simulink model "test_ic_delta_mapping"  (R2025b)
settings: Solver=FixedStepAuto  StartTime=0.0  StopTime=5  FixedStep=50e-6  RelTol=1e-3
undefined symbols (not defined in the file or in its folder): D_201, delta0_201, M_201, Pe_scale, Pm_201, Pm_step_amp_201, Pm_step_t_201, Vmag_201, VSGScale_201, wn_const
libraries: spsControlledVoltageSourceLib x3, spsSeriesRLCBranchLib x3, spsGroundLib x1, spsThreePhasePISectionLineLib x1, spsThreePhaseVIMeasurementLib x1, spsThreePhaseSourceLib x1, spspowerguiLib x1
settings Model: Creator=27443  LastModifiedBy=27443

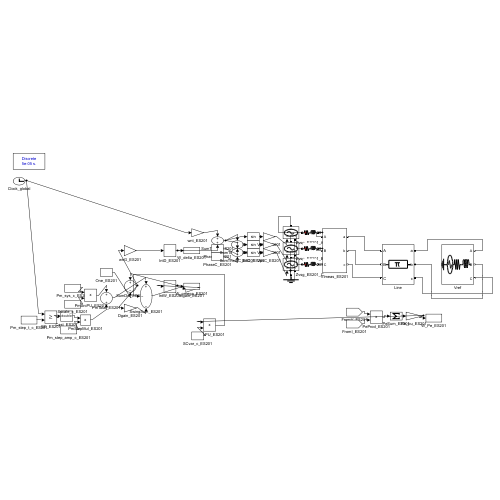
[thumbnail: Simulink's stored preview of the top-level diagram]
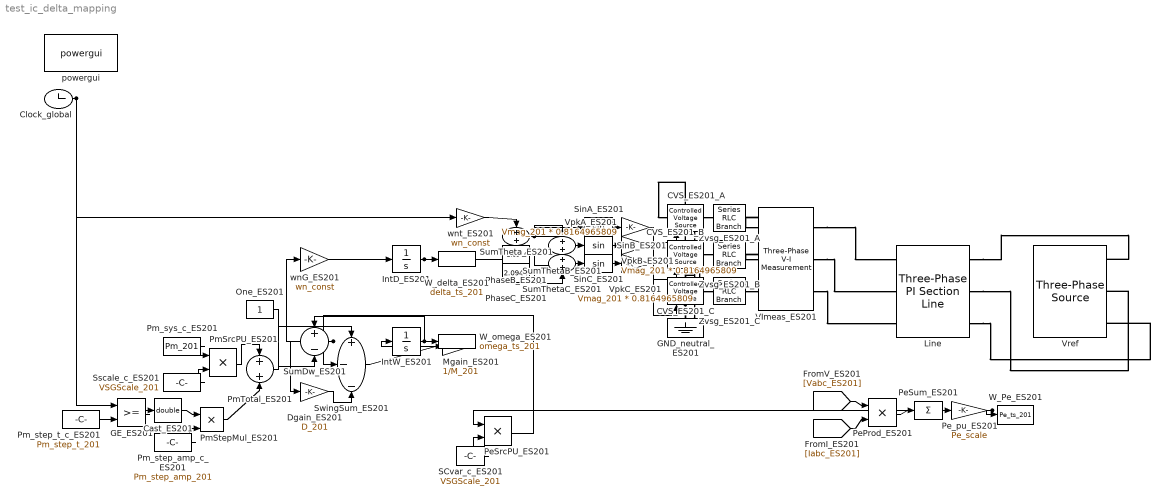
== system test_ic_delta_mapping ==
  CVS_ES201_A : spsControlledVoltageSourceLib/Controlled Voltage Source  Initialize=on  Source_Type=AC  Amplitude=0  Phase=0  Frequency=0  Measurements=None
  CVS_ES201_B : spsControlledVoltageSourceLib/Controlled Voltage Source  Initialize=on  Source_Type=AC  Amplitude=0  Phase=0  Frequency=0  Measurements=None
  CVS_ES201_C : spsControlledVoltageSourceLib/Controlled Voltage Source  Initialize=on  Source_Type=AC  Amplitude=0  Phase=0  Frequency=0  Measurements=None
  Cast_ES201 : DataTypeConversion  OutDataTypeStr=double  SaturateOnIntegerOverflow=off  RndMeth=Floor
  Clock_global : Clock
  Dgain_ES201 : Gain  Gain=D_201
  GE_ES201 : RelationalOperator  OutDataTypeStr=boolean  RndMeth=Simplest  InputSameDT=off
  GND_neutral_ES201 : spsGroundLib/Ground  LConnTagsString=a
  IntD_ES201 : Integrator  InitialCondition=delta0_201
  IntW_ES201 : Integrator  InitialCondition=1
  Line : spsThreePhasePISectionLineLib/Three-Phase PI Section Line  LConnTagsString=a|b|c  RConnTagsString=A|B|C  Length=1  Frequency=50  Resistances=[0.053 0.159]  Inductances=[0.00141 0.00423]  Capacitances=[9e-09 5.4e-09]
  Mgain_ES201 : Gain  Gain=1/M_201
  One_ES201 : Constant
  PeProd_ES201 : Product
  PeSrcPU_ES201 : Product
  PeSum_ES201 : Sum  Inputs=+
  Pe_pu_ES201 : Gain  Gain=Pe_scale
  PhaseB_ES201 : Constant  Value=-2.0944
  PhaseC_ES201 : Constant  Value=2.0944
  PmSrcPU_ES201 : Product
  PmStepMul_ES201 : Product
  PmTotal_ES201 : Sum
  Pm_step_amp_c_ES201 : Constant  Value=Pm_step_amp_201
  Pm_step_t_c_ES201 : Constant  Value=Pm_step_t_201
  Pm_sys_c_ES201 : Constant  Value=Pm_201
  SCvar_c_ES201 : Constant  Value=VSGScale_201
  SinA_ES201 : Trigonometry
  SinB_ES201 : Trigonometry
  SinC_ES201 : Trigonometry
  Sscale_c_ES201 : Constant  Value=VSGScale_201
  SumDw_ES201 : Sum  Inputs=+-
  SumThetaB_ES201 : Sum
  SumThetaC_ES201 : Sum
  SumTheta_ES201 : Sum
  SwingSum_ES201 : Sum  Inputs=+--
  VImeas_ES201 : spsThreePhaseVIMeasurementLib/Three-Phase V-I Measurement  VoltageMeasurement=phase-to-ground  SetLabelV=on  LabelV=Vabc_ES201  Vpu=off  VpuLL=off  CurrentMeasurement=yes  SetLabelI=on  LabelI=Iabc_ES201  Ipu=off  Pbase=100e6  Vbase=500e3  OutputType=Complex  PhasorSimulation=off  PSBequivalent=0
  VpkA_ES201 : Gain  Gain=Vmag_201 * 0.8164965809
  VpkB_ES201 : Gain  Gain=Vmag_201 * 0.8164965809
  VpkC_ES201 : Gain  Gain=Vmag_201 * 0.8164965809
  Vref : spsThreePhaseSourceLib/Three-Phase Source  InternalConnection=Yg  VoltagePhases=off  Voltage=230000  PhaseAngle=0  Voltage_phases=[25e3 25e3 25e3]/sqrt(3)  PhaseAngles_phases=[0 -120 +120]  Frequency=50  NonIdealSource=on  SpecifyImpedance=on  Resistance=0.8929  Inductance=16.58e-3  ShortCircuitLevel=100000e6  BaseVoltage=230000  XRratio=7  BusType=swing  Pref=10e3  Qref=0  Prefabc=[10e3, 10e3, 10e3]  Qrefabc=[0, 0, 0]  Qmin=-inf  Qmax=inf
  W_Pe_ES201 : ToWorkspace  VariableName=Pe_ts_201  SaveFormat=Timeseries  SampleTime=-1
  W_delta_ES201 : ToWorkspace  VariableName=delta_ts_201  SaveFormat=Timeseries  SampleTime=-1
  W_omega_ES201 : ToWorkspace  VariableName=omega_ts_201  SaveFormat=Timeseries  SampleTime=-1
  Zvsg_ES201_A : spsSeriesRLCBranchLib/Series RLC Branch  LConnTagsString=__new0  RConnTagsString=__new0  BranchType=RL  Resistance=0.7935  Inductance=0.25258  SetiL0=off  InitialCurrent=0  Capacitance=1e-6  Setx0=off  InitialVoltage=0  Measurements=None
  Zvsg_ES201_B : spsSeriesRLCBranchLib/Series RLC Branch  LConnTagsString=__new0  RConnTagsString=__new0  BranchType=RL  Resistance=0.7935  Inductance=0.25258  SetiL0=off  InitialCurrent=0  Capacitance=1e-6  Setx0=off  InitialVoltage=0  Measurements=None
  Zvsg_ES201_C : spsSeriesRLCBranchLib/Series RLC Branch  LConnTagsString=__new0  RConnTagsString=__new0  BranchType=RL  Resistance=0.7935  Inductance=0.25258  SetiL0=off  InitialCurrent=0  Capacitance=1e-6  Setx0=off  InitialVoltage=0  Measurements=None
  powergui : spspowerguiLib/powergui  Priority=1  SimulationMode=Discrete  SampleTime=50e-6  frequency=60  Iterations=50  frequencyindice=60  Pbase=100e6  ErrMax=1e-4  UnitsV=kV  UnitsW=MW  buscounter=0  FunctionMessages=off  echomessages=off  EnableUseOfTLC=off  CurrentSourceSwitches=off  DisableSnubberDevices=off  DisableRonSwitches=off  DisableVfSwitches=off  DisplayEquations=off  AutomaticDiscreteSolvers=off  SolverType=Tustin/Backward Euler (TBE)  Interpol=off  ExternalGateDelay=off  methode=off  Ts=100  x0status=blocks  SPID=on  SwTol=0  HookPort=off  NonlinearTolerance=1e-4  nMaxIteration=100  ContinueOnMaxIteration=off  RestoreLinks=warning  ResistiveCurrentMeasurement=off  Frange=[0:2:500]  Ylog=off  Xlog=on  ShowGrid=off  save=off  variable=ZData  structure=0  ZoomFFT=off  StartTime=0.0  cycles=1  DisplayStyle=1  fundamental=60  FreqAxis=off  MaxFrequency=1000  frequencyindicesteady=1  RmsSteady=1  display=off
  wnG_ES201 : Gain  Gain=wn_const
  wnt_ES201 : Gain  Gain=wn_const
  wires:
  Clock_global/1 -> GE_ES201/1, wnt_ES201/1
  Pm_step_t_c_ES201/1 -> GE_ES201/2
  GE_ES201/1 -> Cast_ES201/1
  Cast_ES201/1 -> PmStepMul_ES201/1
  Pm_step_amp_c_ES201/1 -> PmStepMul_ES201/2
  Pm_sys_c_ES201/1 -> PmSrcPU_ES201/1
  Sscale_c_ES201/1 -> PmSrcPU_ES201/2
  PmSrcPU_ES201/1 -> PmTotal_ES201/1
  PmStepMul_ES201/1 -> PmTotal_ES201/2
  IntW_ES201/1 -> SumDw_ES201/1, W_omega_ES201/1
  One_ES201/1 -> SumDw_ES201/2
  SumDw_ES201/1 -> Dgain_ES201/1, wnG_ES201/1
  PmTotal_ES201/1 -> SwingSum_ES201/1
  Dgain_ES201/1 -> SwingSum_ES201/3
  SwingSum_ES201/1 -> Mgain_ES201/1
  Mgain_ES201/1 -> IntW_ES201/1
  wnG_ES201/1 -> IntD_ES201/1
  wnt_ES201/1 -> SumTheta_ES201/1
  IntD_ES201/1 -> SumTheta_ES201/2, W_delta_ES201/1
  SumTheta_ES201/1 -> SumThetaB_ES201/1, SumThetaC_ES201/1, SinA_ES201/1
  PhaseB_ES201/1 -> SumThetaB_ES201/2
  PhaseC_ES201/1 -> SumThetaC_ES201/2
  SumThetaB_ES201/1 -> SinB_ES201/1
  SumThetaC_ES201/1 -> SinC_ES201/1
  SinA_ES201/1 -> VpkA_ES201/1
  SinB_ES201/1 -> VpkB_ES201/1
  SinC_ES201/1 -> VpkC_ES201/1
  VpkA_ES201/1 -> CVS_ES201_A/1
  VpkB_ES201/1 -> CVS_ES201_B/1
  VpkC_ES201/1 -> CVS_ES201_C/1
  [Vabc_ES201] -> PeProd_ES201/1
  [Iabc_ES201] -> PeProd_ES201/2
  PeProd_ES201/1 -> PeSum_ES201/1
  PeSum_ES201/1 -> Pe_pu_ES201/1
  Pe_pu_ES201/1 -> PeSrcPU_ES201/1, W_Pe_ES201/1
  SCvar_c_ES201/1 -> PeSrcPU_ES201/2
  PeSrcPU_ES201/1 -> SwingSum_ES201/2
  connections:
  CVS_ES201_A/LConn1 -- CVS_ES201_B/LConn1 -- GND_neutral_ES201/LConn1 -- CVS_ES201_C/LConn1
  CVS_ES201_A/RConn1 -- Zvsg_ES201_A/LConn1
  CVS_ES201_B/RConn1 -- Zvsg_ES201_B/LConn1
  CVS_ES201_C/RConn1 -- Zvsg_ES201_C/LConn1
  Zvsg_ES201_A/RConn1 -- VImeas_ES201/LConn1
  Zvsg_ES201_B/RConn1 -- VImeas_ES201/LConn2
  Zvsg_ES201_C/RConn1 -- VImeas_ES201/LConn3
  VImeas_ES201/RConn1 -- Line/LConn1
  VImeas_ES201/RConn2 -- Line/LConn2
  VImeas_ES201/RConn3 -- Line/LConn3
  Line/RConn1 -- Vref/RConn1
  Line/RConn2 -- Vref/RConn2
  Line/RConn3 -- Vref/RConn3
